simulink model "My747m14"  (R2021b)
settings: Solver=VariableStepAuto  StartTime=0.0  StopTime=200  RelTol=1e-3
values from neighbouring files (symbols this model uses):
  B = B(:,1:2)    [TwoTankSystem.m]
  K = K_of(:,1:4)    [TwoTankSystem.m]
undefined symbols (not defined in the file or in its folder): A, C
settings Model: Creator=tanzc  LastModifiedBy=tanzc
settings DataIOCC: ReturnWorkspaceOutputs=off

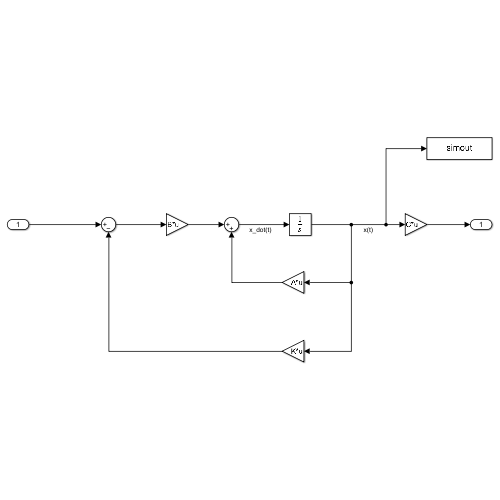
[thumbnail: Simulink's stored preview of the top-level diagram]
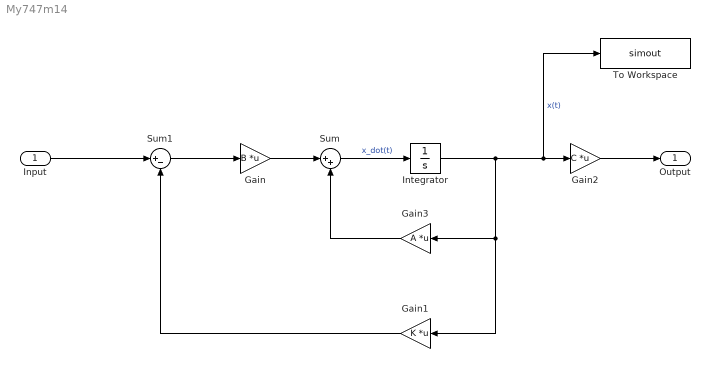
== system My747m14 ==
  Input : Inport  PortDimensions=2
  Gain : Gain  Gain=B  Multiplication=Matrix(K*u)
  Gain1 : Gain  Gain=K  Multiplication=Matrix(K*u)
  Gain2 : Gain  Gain=C  Multiplication=Matrix(K*u)
  Gain3 : Gain  Gain=A  Multiplication=Matrix(K*u)
  Integrator : Integrator
  Sum : Sum  Inputs=|++
  Sum1 : Sum  Inputs=|+-
  To Workspace : ToWorkspace  VariableName=simout  SaveFormat=Timeseries  SampleTime=-1
  Output : Outport
  wires:
  Gain/1 -> Sum/1
  Integrator/1 -> Gain1/1, Gain3/1, To Workspace/1, Gain2/1  "x(t)"
  Sum/1 -> Integrator/1  "x_dot(t)"
  Gain3/1 -> Sum/2
  Sum1/1 -> Gain/1
  Gain2/1 -> Output/1
  Gain1/1 -> Sum1/2
  Input/1 -> Sum1/1
